simulink model "Clutchless_P2_Parallel"  (R2017b)
settings: Solver=FixedStepAuto  StartTime=0.0  StopTime=length(Speed)  FixedStep=0.01  MaxStep=0.01  RelTol=1e-3  EnableMultiTasking=on
PostLoadFcn:
  | , if any(exist('dsrtsu_mdlpostloadfcn', 'file') == [2, 3, 6]), try dsrtsu_mdlpostloadfcn('Execute', bdroot); catch fprintf('Error in PostLoadFcn (dsrtsu_mdlpostloadfcn) for model "%s":\n %s\n', bdroot, lasterr); end, end,
undefined symbols (not defined in the file): Actuators, APP1_OOR, APP2_OOR, APP_Mismatch, Brk_Flt, cal, Chassis, ClutchEngag, Clutchless_HSC, eng, Engine, EngineTorqueReal, EngOverTemp, ENGTRQ_MSMCH_Degraded_CP, ENGTRQ_MSMCH_ErrCritical_CP, ENGTRQ_MSMCH_LimpHome_CP, EngTrqMismatch, ess, ESSOverTemp, g, gb, Grade, KeyPos_Flt, lib_Actuators, lib_Chassis, lib_Clutchless_HSC, lib_EMachine_2017a, lib_Sensors_2017a, LossCAN, Machine, MCUOverTemp, mot, MotDirMismatch, motor_Trq, MotOverTemp, MotTrqMismatch, mph2ms, PRNDL_Flt, RegenFault, rho, Sensors, t_amb, time, tloop, veh, Vehicle
libraries: simulink x96, EC2_libraries x6, autolibmappedmotor x3, powerlib_meascontrol x2, CalculationGallon x1, lib_DCDC x1, lib_Differential x1, lib_HVESS x1, lib_Engine x1, lib_OBC x1, Scope_new x1, lib_Transmission x1
(part 8 of 10)

== system Clutchless_P2_Parallel/Camaro Plant Model/E-Machine/IMG Plant/Electric Machine/Torque Calculation1/max torque  ==
  cmd : Inport
  speed : Inport  Port=2
  Memory : Memory
  Peak trq max - Motoring : Lookup  InputValues=mot.plant.init.regen.trq_max.idx1_spd  Table=mot.plant.init.motor.trq_max.map  LookUpMeth=Interpolation-Use End Values  SaturateOnIntegerOverflow=on
  Peak trq max - Regen : Lookup  InputValues=mot.plant.init.regen.trq_max.idx1_spd  Table=mot.plant.init.regen.trq_max.map  LookUpMeth=Interpolation-Use End Values  SaturateOnIntegerOverflow=on
  Switch1 : Switch  SaturateOnIntegerOverflow=on
  rad/s  to RPM : Gain  Gain=30/pi
  max torque : Outport
  wires:
  Peak trq max - Regen/1 -> Switch1/3
  rad/s  to RPM/1 -> Memory/1
  Memory/1 -> Peak trq max - Regen/1, Peak trq max - Motoring/1
  Switch1/1 -> max torque/1
  cmd/1 -> Switch1/2
  speed/1 -> rad/s  to RPM/1
  Peak trq max - Motoring/1 -> Switch1/1

== system Clutchless_P2_Parallel/Camaro Plant Model/E-Machine/IMG Plant2/Thermal/Motor Thermal/Lower Limit ==
  In1 : Inport
  Constant3 : Constant  Value=Lolimit
  MinMax : MinMax  Function=max  Inputs=2
  Out1 : Outport
  wires:
  MinMax/1 -> Out1/1
  Constant3/1 -> MinMax/2
  In1/1 -> MinMax/1

== system Clutchless_P2_Parallel/Camaro Plant Model/E-Machine/IMG Plant2/Thermal1/MotInv_loop/MCUOverTemp Fault ==
  In1 : Inport
  Gain : Gain  Gain=3
  Switch : Switch  Threshold=1
  Out1 : Outport
  wires:
  Switch/1 -> Out1/1
  Gain/1 -> Switch/1
  [MCUOverTemp] -> Switch/2
  In1/1 -> Gain/1, Switch/3

== system Clutchless_P2_Parallel/Camaro Plant Model/E-Machine/IMG Plant2/Thermal1/MotInv_loop/MotorOverTempFault ==
  In1 : Inport
  Gain : Gain  Gain=2
  Switch1 : Switch  Threshold=1
  Out1 : Outport
  wires:
  Switch1/1 -> Out1/1
  Gain/1 -> Switch1/1
  [MotOverTemp] -> Switch1/2
  In1/1 -> Switch1/3, Gain/1

== system Clutchless_P2_Parallel/Camaro Plant Model/E-Machine/IMG Plant2/Thermal1/Motor Thermal/Lower Limit ==
  In1 : Inport
  Constant3 : Constant  Value=Lolimit
  MinMax : MinMax  Function=max  Inputs=2
  Out1 : Outport
  wires:
  MinMax/1 -> Out1/1
  Constant3/1 -> MinMax/2
  In1/1 -> MinMax/1

== system Clutchless_P2_Parallel/Camaro Plant Model/E-Machine/Soft MCU/Torque Calculation1/max torque /Divide by zero ==
  In1 : Inport
  Compare To Constant : simulink/Logic and Bit Operations/Compare To Constant  relop===  const=0  OutDataTypeStr=boolean
  Constant1 : Constant
  Switch2 : Switch  Criteria=u2 > Threshold
  Out1 : Outport
  wires:
  Constant1/1 -> Switch2/1
  Compare To Constant/1 -> Switch2/2
  In1/1 -> Switch2/3, Compare To Constant/1
  Switch2/1 -> Out1/1

== system Clutchless_P2_Parallel/Camaro Plant Model/E-Machine/Soft MCU/Torque Calculation1/max torque /Heat index ==
  note: Heat index calculation
  cont torque : Inport
  torque : Inport  Port=2
  Abs : Abs  SaturateOnIntegerOverflow=on
  Divide : Subsystem  mask(Divide){}
      mask Display: disp('Divide')
  Heat Energy Factor : Integrator  InitialCondition=-0.3  LimitOutput=on  UpperSaturationLimit=1  LowerSaturationLimit=-0.3
  Heating Constant : Gain  Gain=0.3/mot.plant.init.t_max_trq  SaturateOnIntegerOverflow=on  OutDataTypeStr=Inherit: Same as input  ParamDataTypeStr=Inherit: Same as input
  Saturation : Saturate  UpperLimit=1  LowerLimit=0
  Sum : Sum  Inputs=+-  SaturateOnIntegerOverflow=on  InputSameDT=on  OutDataTypeStr=Inherit: Same as first input
  motor inertia (Nms^2\rad)5 : Constant
  Heat index : Outport
  wires:
  cont torque/1 -> Divide/2(denominator)
  Abs/1 -> Sum/1
  Saturation/1 -> Heat index/1
  motor inertia (Nms^2\rad)5/1 -> Sum/2
  Divide/1(quotient) -> Abs/1
  Sum/1 -> Heating Constant/1
  Heating Constant/1 -> Heat Energy Factor/1
  Heat Energy Factor/1 -> Saturation/1
  torque/1 -> Divide/1(numerator)

== system Clutchless_P2_Parallel/Camaro Plant Model/E-Machine/Soft MCU/Torque Calculation2/max torque /Divide by zero ==
  In1 : Inport
  Compare To Constant : simulink/Logic and Bit Operations/Compare To Constant  relop===  const=0  OutDataTypeStr=boolean
  Constant1 : Constant
  Switch2 : Switch  Criteria=u2 > Threshold
  Out1 : Outport
  wires:
  Constant1/1 -> Switch2/1
  Compare To Constant/1 -> Switch2/2
  In1/1 -> Switch2/3, Compare To Constant/1
  Switch2/1 -> Out1/1

== system Clutchless_P2_Parallel/Camaro Plant Model/E-Machine/Soft MCU/Torque Calculation2/max torque /Heat index ==
  note: Heat index calculation
  cont torque : Inport
  torque : Inport  Port=2
  Abs : Abs  SaturateOnIntegerOverflow=on
  Divide : Subsystem  mask(Divide){}
      mask Display: disp('Divide')
  Heat Energy Factor : Integrator  InitialCondition=-0.3  LimitOutput=on  UpperSaturationLimit=1  LowerSaturationLimit=-0.3
  Heating Constant : Gain  Gain=0.3/mot.plant.init.t_max_trq  SaturateOnIntegerOverflow=on  OutDataTypeStr=Inherit: Same as input  ParamDataTypeStr=Inherit: Same as input
  Saturation : Saturate  UpperLimit=1  LowerLimit=0
  Sum : Sum  Inputs=+-  SaturateOnIntegerOverflow=on  InputSameDT=on  OutDataTypeStr=Inherit: Same as first input
  motor inertia (Nms^2\rad)5 : Constant
  Heat index : Outport
  wires:
  cont torque/1 -> Divide/2(denominator)
  Abs/1 -> Sum/1
  Saturation/1 -> Heat index/1
  motor inertia (Nms^2\rad)5/1 -> Sum/2
  Divide/1(quotient) -> Abs/1
  Sum/1 -> Heating Constant/1
  Heating Constant/1 -> Heat Energy Factor/1
  Heat Energy Factor/1 -> Saturation/1
  torque/1 -> Divide/1(numerator)

== system Clutchless_P2_Parallel/Camaro Plant Model/E-Machine/Soft MCU/Torque Calculation3/max torque /Divide by zero ==
  In1 : Inport
  Compare To Constant : simulink/Logic and Bit Operations/Compare To Constant  relop===  const=0  OutDataTypeStr=boolean
  Constant1 : Constant
  Switch2 : Switch  Criteria=u2 > Threshold
  Out1 : Outport
  wires:
  Constant1/1 -> Switch2/1
  Compare To Constant/1 -> Switch2/2
  In1/1 -> Switch2/3, Compare To Constant/1
  Switch2/1 -> Out1/1

== system Clutchless_P2_Parallel/Camaro Plant Model/E-Machine/Soft MCU/Torque Calculation3/max torque /Heat index ==
  note: Heat index calculation
  cont torque : Inport
  torque : Inport  Port=2
  Abs : Abs  ZeroCross=off  SaturateOnIntegerOverflow=on
  Divide : Subsystem  mask(Divide){}
      mask Display: disp('Divide')
  Heat Energy Factor : Integrator  InitialCondition=-0.3  LimitOutput=on  UpperSaturationLimit=1  LowerSaturationLimit=-0.3  ZeroCross=off
  Heating Constant : Gain  Gain=0.3/mot.plant.init.t_max_trq  SaturateOnIntegerOverflow=on  OutDataTypeStr=Inherit: Same as input  ParamDataTypeStr=Inherit: Same as input
  Saturation : Saturate  UpperLimit=1  LowerLimit=0  ZeroCross=off
  Sum : Sum  Inputs=+-  SaturateOnIntegerOverflow=on  InputSameDT=on  OutDataTypeStr=Inherit: Same as first input
  motor inertia (Nms^2\rad)5 : Constant
  Heat index : Outport
  wires:
  cont torque/1 -> Divide/2(denominator)
  Abs/1 -> Sum/1
  Saturation/1 -> Heat index/1
  motor inertia (Nms^2\rad)5/1 -> Sum/2
  Divide/1(quotient) -> Abs/1
  Sum/1 -> Heating Constant/1
  Heating Constant/1 -> Heat Energy Factor/1
  Heat Energy Factor/1 -> Saturation/1
  torque/1 -> Divide/1(numerator)

== system Clutchless_P2_Parallel/Clutchless_HSC/HSC/Camaro Fault Detection/Component Diagnostic/Engine Component Diagnostic/Override  engTrqCmd ==
  note: This subsystem is used to override the model value of a signal to a constant value
  note: Override Switch Subsystem
  In1 : Inport
  Constant : Constant  Value=50
  Multiport Switch : MultiPortSwitch  DataPortOrder=Zero-based contiguous  Inputs=2  zeroidx=on
  Signal Override Switch 0 = Use Model 1 = Use Constant : Constant
  Out1 : Outport
  wires:
  Signal Override Switch 0 = Use Model 1 = Use Constant/1 -> Multiport Switch/1
  In1/1 -> Multiport Switch/2
  Multiport Switch/1 -> Out1/1
  Constant/1 -> Multiport Switch/3

== system Clutchless_P2_Parallel/Clutchless_HSC/HSC/Camaro Fault Detection/Component Diagnostic/Engine Component Diagnostic/TorqMismatch Detection ==
  In1 : Inport
  In2 : Inport  Port=2
  In3 : Inport  Port=3
  Abs : Abs
  Add : Sum  Inputs=+-
  Bus Creator : BusCreator  Inputs=3
  Constant : Constant  Value=cal.ENGTRQ_MSMCH.ErrCritical_CP
  Constant1 : Constant  Value=50
  Constant2 : Constant  Value=cal.ENGTRQ_MSMCH.Degraded_CP
  Constant3 : Constant  Value=cal.ENGTRQ_MSMCH.LimpHome_CP
  Constant4 : Constant  Value=0
  Constant5 : Constant  Value=0
  Constant6 : Constant  Value=0
  Data Type Conversion : DataTypeConversion  OutDataTypeStr=boolean
  Data Type Conversion1 : DataTypeConversion  OutDataTypeStr=boolean
  Data Type Conversion2 : DataTypeConversion  OutDataTypeStr=boolean
  Relational Operator : RelationalOperator  OutDataTypeStr=boolean  RndMeth=Nearest
  Relational Operator1 : RelationalOperator  Operator=>  OutDataTypeStr=boolean  RndMeth=Nearest
  Relational Operator2 : RelationalOperator  Operator=>  OutDataTypeStr=boolean  RndMeth=Nearest
  Switch : Switch  Threshold=1
  Terminator{,1..3} (4 alike) : Terminator
  Unit Delay : UnitDelay  Commented=through  SampleTime=-1
  Unit Delay1 : UnitDelay  Commented=through  SampleTime=-1
  "Zero " : Constant  Value=0
  Eng_Torque_Mismch : Outport
  wires:
  Constant1/1 -> Terminator3/1
  In1/1 -> Unit Delay/1
  In2/1 -> Unit Delay1/1
  "Zero "/1 -> Switch/3
  In3/1 -> Switch/2
  Unit Delay/1 -> Add/1
  Constant/1 -> Relational Operator/2
  Add/1 -> Abs/1
  Relational Operator/1 -> Switch/1
  Switch/1 -> Relational Operator2/1, Relational Operator1/1, Terminator/1  "Eng_Torque_Mismch_Critical"
  Constant2/1 -> Relational Operator1/2
  Constant3/1 -> Relational Operator2/2
  Relational Operator1/1 -> Terminator1/1  "Eng_Torque_Mismch_Degrad"
  Relational Operator2/1 -> Terminator2/1  "Eng_Torque_Mismch_Limp"
  Bus Creator/1 -> Eng_Torque_Mismch/1
  Unit Delay1/1 -> Add/2
  Abs/1 -> Relational Operator/1
  Constant4/1 -> Data Type Conversion/1  "Eng_Torque_Mismch_Critical"
  Constant6/1 -> Data Type Conversion2/1  "Eng_Torque_Mismch_Limp"
  Constant5/1 -> Data Type Conversion1/1  "Eng_Torque_Mismch_Degrad"
  Data Type Conversion/1 -> Bus Creator/1  "Eng_Torque_Mismch_Critical"
  Data Type Conversion1/1 -> Bus Creator/2  "Eng_Torque_Mismch_Degrad"
  Data Type Conversion2/1 -> Bus Creator/3  "Eng_Torque_Mismch_Limp"

== system Clutchless_P2_Parallel/Clutchless_HSC/HSC/Camaro Fault Detection/Input Conversions/BMS_Conversions/Override  BMS_gdf 0_1 ==
  note: Override Switch Subsystem
  note: This subsystem is used to override the model value of a signal to a constant value
  In1 : Inport
  Multiport Switch : MultiPortSwitch  DataPortOrder=Zero-based contiguous  Inputs=2  zeroidx=on
  Override Value : Constant  Value=0  OutDataTypeStr=double
  Signal Override Switch 0 = Use Model 1 = Use Constant : Constant
  Out1 : Outport
  wires:
  Override Value/1 -> Multiport Switch/3
  Multiport Switch/1 -> Out1/1
  In1/1 -> Multiport Switch/2
  Signal Override Switch 0 = Use Model 1 = Use Constant/1 -> Multiport Switch/1

== system Clutchless_P2_Parallel/Clutchless_HSC/HSC/Camaro Fault Detection/Input Conversions/BMS_Conversions/Override  closeContactorsCmd ==
  note: This subsystem is used to override the model value of a signal to a constant value
  note: Override Switch Subsystem
  In1 : Inport
  Multiport Switch : MultiPortSwitch  DataPortOrder=Zero-based contiguous  Inputs=2  zeroidx=on
  Override Value : Constant  Value=0  OutDataTypeStr=double
  Signal Override Switch 0 = Use Model 1 = Use Constant : Constant  Value=0
  Out1 : Outport
  wires:
  Signal Override Switch 0 = Use Model 1 = Use Constant/1 -> Multiport Switch/1
  In1/1 -> Multiport Switch/2
  Multiport Switch/1 -> Out1/1
  Override Value/1 -> Multiport Switch/3

== system Clutchless_P2_Parallel/Clutchless_HSC/HSC/Camaro Fault Detection/Input Conversions/BMS_Conversions/Override  contactorsClsd ==
  note: This subsystem is used to override the model value of a signal to a constant value
  note: Override Switch Subsystem
  In1 : Inport
  Multiport Switch : MultiPortSwitch  DataPortOrder=Zero-based contiguous  Inputs=2  zeroidx=on
  Override Value : Constant  Value=0  OutDataTypeStr=double
  Signal Override Switch 0 = Use Model 1 = Use Constant : Constant  Value=0
  Out1 : Outport
  wires:
  Signal Override Switch 0 = Use Model 1 = Use Constant/1 -> Multiport Switch/1
  In1/1 -> Multiport Switch/2
  Multiport Switch/1 -> Out1/1
  Override Value/1 -> Multiport Switch/3

== system Clutchless_P2_Parallel/Clutchless_HSC/HSC/Camaro Fault Detection/Input Conversions/BMS_Conversions/Override  essCur_A ==
  note: Override Switch Subsystem
  note: This subsystem is used to override the model value of a signal to a constant value
  In1 : Inport
  Multiport Switch : MultiPortSwitch  DataPortOrder=Zero-based contiguous  Inputs=2  zeroidx=on
  Override Value : Constant  Value=0  OutDataTypeStr=double
  Signal Override Switch 0 = Use Model 1 = Use Constant : Constant  Value=0
  Out1 : Outport
  wires:
  Override Value/1 -> Multiport Switch/3
  Multiport Switch/1 -> Out1/1
  In1/1 -> Multiport Switch/2
  Signal Override Switch 0 = Use Model 1 = Use Constant/1 -> Multiport Switch/1

== system Clutchless_P2_Parallel/Clutchless_HSC/HSC/Camaro Fault Detection/Input Conversions/BMS_Conversions/Override  essSOC_0_1 ==
  note: This subsystem is used to override the model value of a signal to a constant value
  note: Override Switch Subsystem
  In1 : Inport
  Multiport Switch : MultiPortSwitch  DataPortOrder=Zero-based contiguous  Inputs=2  zeroidx=on
  Override Value : Constant  Value=0  OutDataTypeStr=double
  Signal Override Switch 0 = Use Model 1 = Use Constant : Constant  Value=0
  Out1 : Outport
  wires:
  Signal Override Switch 0 = Use Model 1 = Use Constant/1 -> Multiport Switch/1
  In1/1 -> Multiport Switch/2
  Multiport Switch/1 -> Out1/1
  Override Value/1 -> Multiport Switch/3

== system Clutchless_P2_Parallel/Clutchless_HSC/HSC/Camaro Fault Detection/Input Conversions/BMS_Conversions/Override  essTemp_C ==
  note: This subsystem is used to override the model value of a signal to a constant value
  note: Override Switch Subsystem
  In1 : Inport
  Multiport Switch : MultiPortSwitch  DataPortOrder=Zero-based contiguous  Inputs=2  zeroidx=on
  Override Value : Constant  Value=0  OutDataTypeStr=double
  Signal Override Switch 0 = Use Model 1 = Use Constant : Constant
  Out1 : Outport
  wires:
  Signal Override Switch 0 = Use Model 1 = Use Constant/1 -> Multiport Switch/1
  In1/1 -> Multiport Switch/2
  Multiport Switch/1 -> Out1/1
  Override Value/1 -> Multiport Switch/3

== system Clutchless_P2_Parallel/Clutchless_HSC/HSC/Camaro Fault Detection/Input Conversions/BMS_Conversions/Override  hvBattVolt_V ==
  note: This subsystem is used to override the model value of a signal to a constant value
  note: Override Switch Subsystem
  In1 : Inport
  Multiport Switch : MultiPortSwitch  DataPortOrder=Zero-based contiguous  Inputs=2  zeroidx=on
  Override Value : Constant  Value=0  OutDataTypeStr=double
  Signal Override Switch 0 = Use Model 1 = Use Constant : Constant  Value=0
  Out1 : Outport
  wires:
  Signal Override Switch 0 = Use Model 1 = Use Constant/1 -> Multiport Switch/1
  In1/1 -> Multiport Switch/2
  Multiport Switch/1 -> Out1/1
  Override Value/1 -> Multiport Switch/3

== system Clutchless_P2_Parallel/Clutchless_HSC/HSC/Camaro Fault Detection/Input Conversions/BMS_Conversions/Override  hvBusVolt_V ==
  note: Override Switch Subsystem
  note: This subsystem is used to override the model value of a signal to a constant value
  In1 : Inport
  Multiport Switch : MultiPortSwitch  DataPortOrder=Zero-based contiguous  Inputs=2  zeroidx=on
  Override Value : Constant  Value=0  OutDataTypeStr=double
  Signal Override Switch 0 = Use Model 1 = Use Constant : Constant  Value=0
  Out1 : Outport
  wires:
  Override Value/1 -> Multiport Switch/3
  Multiport Switch/1 -> Out1/1
  In1/1 -> Multiport Switch/2
  Signal Override Switch 0 = Use Model 1 = Use Constant/1 -> Multiport Switch/1

== system Clutchless_P2_Parallel/Clutchless_HSC/HSC/Camaro Fault Detection/Input Conversions/BMS_Conversions/Override  rollingAliveCnt [1_3] ==
  note: Override Switch Subsystem
  note: This subsystem is used to override the model value of a signal to a constant value
  In1 : Inport
  Multiport Switch : MultiPortSwitch  DataPortOrder=Zero-based contiguous  Inputs=2  zeroidx=on
  Override Value : Constant  Value=0  OutDataTypeStr=double
  Signal Override Switch 0 = Use Model 1 = Use Constant : Constant  Value=0
  Out1 : Outport
  wires:
  Override Value/1 -> Multiport Switch/3
  Multiport Switch/1 -> Out1/1
  In1/1 -> Multiport Switch/2
  Signal Override Switch 0 = Use Model 1 = Use Constant/1 -> Multiport Switch/1

== system Clutchless_P2_Parallel/Clutchless_HSC/HSC/Camaro Fault Detection/Input Conversions/BMS_Conversions/Override Fehler_HS_offen ==
  note: This subsystem is used to override the model value of a signal to a constant value
  note: Override Switch Subsystem
  In1 : Inport
  Multiport Switch : MultiPortSwitch  DataPortOrder=Zero-based contiguous  Inputs=2  zeroidx=on
  Override Value : Constant  Value=0  OutDataTypeStr=double
  Signal Override Switch 0 = Use Model 1 = Use Constant : Constant
  Out1 : Outport
  wires:
  Signal Override Switch 0 = Use Model 1 = Use Constant/1 -> Multiport Switch/1
  In1/1 -> Multiport Switch/2
  Multiport Switch/1 -> Out1/1
  Override Value/1 -> Multiport Switch/3

== system Clutchless_P2_Parallel/Clutchless_HSC/HSC/Camaro Fault Detection/Input Conversions/BMS_Conversions/Override Fehler_HS_verschweisst ==
  note: Override Switch Subsystem
  note: This subsystem is used to override the model value of a signal to a constant value
  In1 : Inport
  Multiport Switch : MultiPortSwitch  DataPortOrder=Zero-based contiguous  Inputs=2  zeroidx=on
  Override Value : Constant  Value=0  OutDataTypeStr=double
  Signal Override Switch 0 = Use Model 1 = Use Constant : Constant
  Out1 : Outport
  wires:
  Override Value/1 -> Multiport Switch/3
  Multiport Switch/1 -> Out1/1
  In1/1 -> Multiport Switch/2
  Signal Override Switch 0 = Use Model 1 = Use Constant/1 -> Multiport Switch/1

== system Clutchless_P2_Parallel/Clutchless_HSC/HSC/Camaro Fault Detection/Input Conversions/DriverInput_Conversions/Override  KeyPos [0_3] ==
  note: Override Switch Subsystem
  note: This subsystem is used to override the model value of a signal to a constant value
  In1 : Inport
  Multiport Switch : MultiPortSwitch  DataPortOrder=Zero-based contiguous  Inputs=2  zeroidx=on
  Override Value : Constant  Value=0  OutDataTypeStr=double
  Signal Override Switch 0 = Use Model 1 = Use Constant : Constant  Value=0
  Out1 : Outport
  wires:
  Override Value/1 -> Multiport Switch/3
  Multiport Switch/1 -> Out1/1
  In1/1 -> Multiport Switch/2
  Signal Override Switch 0 = Use Model 1 = Use Constant/1 -> Multiport Switch/1

== system Clutchless_P2_Parallel/Clutchless_HSC/HSC/Camaro Fault Detection/Input Conversions/DriverInput_Conversions/Override APP (%) ==
  note: Override Switch Subsystem
  note: This subsystem is used to override the model value of a signal to a constant value
  In1 : Inport
  Multiport Switch : MultiPortSwitch  DataPortOrder=Zero-based contiguous  Inputs=2  zeroidx=on
  Override Value : Constant  Value=0  OutDataTypeStr=double
  Signal Override Switch 0 = Use Model 1 = Use Constant : Constant  Value=0
  Out1 : Outport
  wires:
  Override Value/1 -> Multiport Switch/3
  Multiport Switch/1 -> Out1/1
  In1/1 -> Multiport Switch/2
  Signal Override Switch 0 = Use Model 1 = Use Constant/1 -> Multiport Switch/1

== system Clutchless_P2_Parallel/Clutchless_HSC/HSC/Camaro Fault Detection/Input Conversions/DriverInput_Conversions/Override APP (%)1 ==
  note: This subsystem is used to override the model value of a signal to a constant value
  note: Override Switch Subsystem
  In1 : Inport
  Multiport Switch : MultiPortSwitch  DataPortOrder=Zero-based contiguous  Inputs=2  zeroidx=on
  Override Value : Constant  Value=0  OutDataTypeStr=double
  Signal Override Switch 0 = Use Model 1 = Use Constant : Constant  Value=0
  Out1 : Outport
  wires:
  Signal Override Switch 0 = Use Model 1 = Use Constant/1 -> Multiport Switch/1
  In1/1 -> Multiport Switch/2
  Multiport Switch/1 -> Out1/1
  Override Value/1 -> Multiport Switch/3

== system Clutchless_P2_Parallel/Clutchless_HSC/HSC/Camaro Fault Detection/Input Conversions/DriverInput_Conversions/Override BPP (%) ==
  note: This subsystem is used to override the model value of a signal to a constant value
  note: Override Switch Subsystem
  In1 : Inport
  Multiport Switch : MultiPortSwitch  DataPortOrder=Zero-based contiguous  Inputs=2  zeroidx=on
  Override Value : Constant  Value=0  OutDataTypeStr=double
  Signal Override Switch 0 = Use Model 1 = Use Constant : Constant  Value=0
  Out1 : Outport
  wires:
  Signal Override Switch 0 = Use Model 1 = Use Constant/1 -> Multiport Switch/1
  In1/1 -> Multiport Switch/2
  Multiport Switch/1 -> Out1/1
  Override Value/1 -> Multiport Switch/3

== system Clutchless_P2_Parallel/Clutchless_HSC/HSC/Camaro Fault Detection/Input Conversions/DriverInput_Conversions/Override PRNDL ==
  note: Override Switch Subsystem
  note: This subsystem is used to override the model value of a signal to a constant value
  In1 : Inport
  Multiport Switch : MultiPortSwitch  DataPortOrder=Zero-based contiguous  Inputs=2  zeroidx=on
  Override Value : Constant  Value=0  OutDataTypeStr=double
  Signal Override Switch 0 = Use Model 1 = Use Constant : Constant  Value=0
  Out1 : Outport
  wires:
  Override Value/1 -> Multiport Switch/3
  Multiport Switch/1 -> Out1/1
  In1/1 -> Multiport Switch/2
  Signal Override Switch 0 = Use Model 1 = Use Constant/1 -> Multiport Switch/1

== system Clutchless_P2_Parallel/Clutchless_HSC/HSC/Camaro Fault Detection/Input Conversions/DriverInput_Conversions/Override Regen ==
  note: Override Switch Subsystem
  note: This subsystem is used to override the model value of a signal to a constant value
  In1 : Inport
  Multiport Switch : MultiPortSwitch  DataPortOrder=Zero-based contiguous  Inputs=2  zeroidx=on
  Override Value : Constant  Value=0  OutDataTypeStr=double
  Signal Override Switch 0 = Use Model 1 = Use Constant : Constant  Value=0
  Out1 : Outport
  wires:
  Override Value/1 -> Multiport Switch/3
  Multiport Switch/1 -> Out1/1
  In1/1 -> Multiport Switch/2
  Signal Override Switch 0 = Use Model 1 = Use Constant/1 -> Multiport Switch/1

== system Clutchless_P2_Parallel/Clutchless_HSC/HSC/Camaro Fault Detection/Input Conversions/DriverInput_Conversions/Override V [mph] ==
  note: This subsystem is used to override the model value of a signal to a constant value
  note: Override Switch Subsystem
  In1 : Inport
  Multiport Switch : MultiPortSwitch  DataPortOrder=Zero-based contiguous  Inputs=2  zeroidx=on
  Override Value : Constant  Value=0  OutDataTypeStr=double
  Signal Override Switch 0 = Use Model 1 = Use Constant : Constant  Value=0
  Out1 : Outport
  wires:
  Signal Override Switch 0 = Use Model 1 = Use Constant/1 -> Multiport Switch/1
  In1/1 -> Multiport Switch/2
  Multiport Switch/1 -> Out1/1
  Override Value/1 -> Multiport Switch/3

== system Clutchless_P2_Parallel/Clutchless_HSC/HSC/Camaro Fault Detection/Input Conversions/ECM_Conversions/Override  ECMTrqCmd_Nm ==
  note: This subsystem is used to override the model value of a signal to a constant value
  note: Override Switch Subsystem
  In1 : Inport
  Multiport Switch : MultiPortSwitch  DataPortOrder=Zero-based contiguous  Inputs=2  zeroidx=on
  Override Value : Constant  Value=0  OutDataTypeStr=double
  Signal Override Switch 0 = Use Model 1 = Use Constant : Constant  Value=0
  Out1 : Outport
  wires:
  Signal Override Switch 0 = Use Model 1 = Use Constant/1 -> Multiport Switch/1
  In1/1 -> Multiport Switch/2
  Multiport Switch/1 -> Out1/1
  Override Value/1 -> Multiport Switch/3

== system Clutchless_P2_Parallel/Clutchless_HSC/HSC/Camaro Fault Detection/Input Conversions/ECM_Conversions/Override  ECMrollingAliveCnt ==
  note: Override Switch Subsystem
  note: This subsystem is used to override the model value of a signal to a constant value
  In1 : Inport
  Multiport Switch : MultiPortSwitch  DataPortOrder=Zero-based contiguous  Inputs=2  zeroidx=on
  Override Value : Constant  Value=0  OutDataTypeStr=double
  Signal Override Switch 0 = Use Model 1 = Use Constant : Constant  Value=0
  Out1 : Outport
  wires:
  Override Value/1 -> Multiport Switch/3
  Multiport Switch/1 -> Out1/1
  In1/1 -> Multiport Switch/2
  Signal Override Switch 0 = Use Model 1 = Use Constant/1 -> Multiport Switch/1

== system Clutchless_P2_Parallel/Clutchless_HSC/HSC/Camaro Fault Detection/Input Conversions/ECM_Conversions/Override  EngActStdyStTorq_Nm ==
  note: Override Switch Subsystem
  note: This subsystem is used to override the model value of a signal to a constant value
  In1 : Inport
  Multiport Switch : MultiPortSwitch  DataPortOrder=Zero-based contiguous  Inputs=2  zeroidx=on
  Override Value : Constant  Value=0  OutDataTypeStr=double
  Signal Override Switch 0 = Use Model 1 = Use Constant : Constant  Value=0
  Out1 : Outport
  wires:
  Override Value/1 -> Multiport Switch/3
  Multiport Switch/1 -> Out1/1
  In1/1 -> Multiport Switch/2
  Signal Override Switch 0 = Use Model 1 = Use Constant/1 -> Multiport Switch/1

== system Clutchless_P2_Parallel/Clutchless_HSC/HSC/Camaro Fault Detection/Input Conversions/ECM_Conversions/Override  EngRunAtv ==
  note: This subsystem is used to override the model value of a signal to a constant value
  note: Override Switch Subsystem
  In1 : Inport
  Multiport Switch : MultiPortSwitch  DataPortOrder=Zero-based contiguous  Inputs=2  zeroidx=on
  Override Value : Constant  Value=0  OutDataTypeStr=double
  Signal Override Switch 0 = Use Model 1 = Use Constant : Constant  Value=0
  Out1 : Outport
  wires:
  Signal Override Switch 0 = Use Model 1 = Use Constant/1 -> Multiport Switch/1
  In1/1 -> Multiport Switch/2
  Multiport Switch/1 -> Out1/1
  Override Value/1 -> Multiport Switch/3

== system Clutchless_P2_Parallel/Clutchless_HSC/HSC/Camaro Fault Detection/Input Conversions/ECM_Conversions/Override  EngineSpeed_rpm ==
  note: This subsystem is used to override the model value of a signal to a constant value
  note: Override Switch Subsystem
  In1 : Inport
  Multiport Switch : MultiPortSwitch  DataPortOrder=Zero-based contiguous  Inputs=2  zeroidx=on
  Override Value : Constant  Value=0  OutDataTypeStr=double
  Signal Override Switch 0 = Use Model 1 = Use Constant : Constant  Value=0
  Out1 : Outport
  wires:
  Signal Override Switch 0 = Use Model 1 = Use Constant/1 -> Multiport Switch/1
  In1/1 -> Multiport Switch/2
  Multiport Switch/1 -> Out1/1
  Override Value/1 -> Multiport Switch/3

== system Clutchless_P2_Parallel/Clutchless_HSC/HSC/Camaro Fault Detection/Input Conversions/ECM_Conversions/Override  Engine_Temp[DegC] ==
  note: Override Switch Subsystem
  note: This subsystem is used to override the model value of a signal to a constant value
  In1 : Inport
  Multiport Switch : MultiPortSwitch  DataPortOrder=Zero-based contiguous  Inputs=2  zeroidx=on
  Override Value : Constant  Value=0  OutDataTypeStr=double
  Signal Override Switch 0 = Use Model 1 = Use Constant : Constant  Value=0
  Out1 : Outport
  wires:
  Override Value/1 -> Multiport Switch/3
  Multiport Switch/1 -> Out1/1
  In1/1 -> Multiport Switch/2
  Signal Override Switch 0 = Use Model 1 = Use Constant/1 -> Multiport Switch/1

== system Clutchless_P2_Parallel/Clutchless_HSC/HSC/Camaro Fault Detection/Input Conversions/TCM_Conversions/Override  LockupCmd ==
  note: This subsystem is used to override the model value of a signal to a constant value
  note: Override Switch Subsystem
  In1 : Inport
  Multiport Switch : MultiPortSwitch  DataPortOrder=Zero-based contiguous  Inputs=2  zeroidx=on
  Override Value : Constant  Value=0  OutDataTypeStr=double
  Signal Override Switch 0 = Use Model 1 = Use Constant : Constant  Value=0
  Out1 : Outport
  wires:
  Signal Override Switch 0 = Use Model 1 = Use Constant/1 -> Multiport Switch/1
  In1/1 -> Multiport Switch/2
  Multiport Switch/1 -> Out1/1
  Override Value/1 -> Multiport Switch/3

== system Clutchless_P2_Parallel/Clutchless_HSC/HSC/Camaro Fault Detection/Input Conversions/TCM_Conversions/Override  LvrPosTrnsShft  ==
  note: This subsystem is used to override the model value of a signal to a constant value
  note: Override Switch Subsystem
  In1 : Inport
  Multiport Switch : MultiPortSwitch  DataPortOrder=Zero-based contiguous  Inputs=2  zeroidx=on
  Override Value : Constant  Value=0  OutDataTypeStr=double
  Signal Override Switch 0 = Use Model 1 = Use Constant : Constant  Value=0
  Out1 : Outport
  wires:
  Signal Override Switch 0 = Use Model 1 = Use Constant/1 -> Multiport Switch/1
  In1/1 -> Multiport Switch/2
  Multiport Switch/1 -> Out1/1
  Override Value/1 -> Multiport Switch/3

== system Clutchless_P2_Parallel/Clutchless_HSC/HSC/Camaro Fault Detection/Input Conversions/TCM_Conversions/Override  TransEstGear ==
  note: This subsystem is used to override the model value of a signal to a constant value
  note: Override Switch Subsystem
  In1 : Inport
  Multiport Switch : MultiPortSwitch  DataPortOrder=Zero-based contiguous  Inputs=2  zeroidx=on
  Override Value : Constant  Value=0  OutDataTypeStr=double
  Signal Override Switch 0 = Use Model 1 = Use Constant : Constant  Value=0
  Out1 : Outport
  wires:
  Signal Override Switch 0 = Use Model 1 = Use Constant/1 -> Multiport Switch/1
  In1/1 -> Multiport Switch/2
  Multiport Switch/1 -> Out1/1
  Override Value/1 -> Multiport Switch/3

== system Clutchless_P2_Parallel/Clutchless_HSC/HSC/Camaro Fault Detection/Input Conversions/TCM_Conversions/Override  rollingAliveCnt [123] ==
  note: This subsystem is used to override the model value of a signal to a constant value
  note: Override Switch Subsystem
  In1 : Inport
  Multiport Switch : MultiPortSwitch  DataPortOrder=Zero-based contiguous  Inputs=2  zeroidx=on
  Override Value : Constant  Value=0  OutDataTypeStr=double
  Signal Override Switch 0 = Use Model 1 = Use Constant : Constant  Value=0
  Out1 : Outport
  wires:
  Signal Override Switch 0 = Use Model 1 = Use Constant/1 -> Multiport Switch/1
  In1/1 -> Multiport Switch/2
  Multiport Switch/1 -> Out1/1
  Override Value/1 -> Multiport Switch/3

== system Clutchless_P2_Parallel/Clutchless_HSC/HSC/Camaro Fault Detection/Input Conversions/TCM_Conversions/TCM_RollinAliveCounter ==
  Constant : Constant  Value=0
  Constant8 : Constant
  Rolling Alive Counter1 : Stateflow chart  TreatAsAtomicUnit=on
  Switch1 : Switch  Criteria=u2 > Threshold
  Out1 : Outport
  wires:
  Constant/1 -> [TCM_CAN_fault]
  Switch1/1 -> Out1/1  "TCMRollingAliveCnt [0 1 2 3]"
  [TCM_CAN_fault] -> Switch1/2
  Rolling Alive Counter1/1(RollingAliveCnt) -> Switch1/3
  Constant8/1 -> Switch1/1

== system Clutchless_P2_Parallel/Clutchless_HSC/HSC/Camaro Fault Detection/Signal Diagnostic/Driver Signal Diagnostic/APP_Crosscheck ==
  In1 : Inport
  In2 : Inport  Port=2
  Abs : Abs
  Compare To Constant : simulink/Logic and Bit Operations/Compare To Constant  relop=<=  const=0.5  OutDataTypeStr=boolean
  Sum : Sum  Inputs=+-
  Out1 : Outport
  wires:
  Sum/1 -> Abs/1
  Abs/1 -> Compare To Constant/1
  In1/1 -> Sum/1
  In2/1 -> Sum/2
  Compare To Constant/1 -> Out1/1  "Drv_APP_Agree"

== system Clutchless_P2_Parallel/Clutchless_HSC/HSC/Camaro Fault Detection/Signal Diagnostic/Driver Signal Diagnostic/BrakeFailureDetection ==
  BPP : Inport
  VehSpeed : Inport  Port=2
  Trigger : TriggerPort  VariantControl=Variant  PortDimensions=1
  Chart : Stateflow chart  Commented=on  TreatAsAtomicUnit=on
  Compare To Constant : simulink/Logic and Bit Operations/Compare To Constant  relop=>  const=0  OutDataTypeStr=boolean
  Compare To Constant1 : simulink/Logic and Bit Operations/Compare To Constant  relop=>  const=0.5  OutDataTypeStr=boolean
  Detect Change : simulink/Logic and Bit Operations/Detect Change  vinit=0  InputProcessing=Inherited  OutDataTypeStr=boolean
  Detect Increase : simulink/Logic and Bit Operations/Detect Increase  vinit=0.0  InputProcessing=Inherited  OutDataTypeStr=boolean
  Logical Operator : Logic  Operator=NOT  AllPortsSameDT=off  OutDataTypeStr=boolean
  Logical Operator1 : Logic  AllPortsSameDT=off  OutDataTypeStr=boolean
  Logical Operator2 : Logic  Operator=OR  AllPortsSameDT=off  OutDataTypeStr=boolean
  Logical Operator3 : Logic  AllPortsSameDT=off  OutDataTypeStr=boolean
  Unit Delay : UnitDelay  SampleTime=-1
  Unit Delay1 : UnitDelay  SampleTime=-1
  DecelFail : Outport
  wires:
  VehSpeed/1 -> Unit Delay1/1, Detect Change/1, Detect Increase/1
  Detect Change/1 -> Logical Operator/1
  Compare To Constant/1 -> Logical Operator1/1
  Compare To Constant1/1 -> Logical Operator1/2
  BPP/1 -> Unit Delay/1
  Logical Operator1/1 -> Logical Operator3/1
  Detect Increase/1 -> Logical Operator2/1  "Increase"
  Logical Operator/1 -> Logical Operator2/2  "Unchange"
  Unit Delay/1 -> Compare To Constant/1
  Unit Delay1/1 -> Compare To Constant1/1
  Logical Operator2/1 -> Logical Operator3/2
  Logical Operator3/1 -> DecelFail/1

== system Clutchless_P2_Parallel/Clutchless_HSC/HSC/Camaro Fault Detection/Signal Diagnostic/Driver Signal Diagnostic/Latch ==
  In1 : Inport
  In2 : Inport  Port=2
  Memory : Memory
  NOT : Logic  Operator=NOT  OutDataTypeStr=boolean
  OR : Logic  OutDataTypeStr=boolean
  OR1 : Logic  Operator=OR  OutDataTypeStr=boolean
  Drv_APP_Agree : Outport
  wires:
  In1/1 -> OR1/1
  OR/1 -> OR1/2
  OR1/1 -> Drv_APP_Agree/1, Memory/1
  NOT/1 -> OR/1
  Memory/1 -> OR/2
  In2/1 -> NOT/1

== system Clutchless_P2_Parallel/Clutchless_HSC/HSC/Camaro Fault Detection/Signal Diagnostic/Driver Signal Diagnostic/Latch1 ==
  In1 : Inport
  In2 : Inport  Port=2
  Memory : Memory
  NOT : Logic  Operator=NOT  OutDataTypeStr=boolean
  OR : Logic  OutDataTypeStr=boolean
  OR1 : Logic  Operator=OR  OutDataTypeStr=boolean
  Out1 : Outport
  wires:
  In2/1 -> NOT/1
  Memory/1 -> OR/2
  NOT/1 -> OR/1
  OR1/1 -> Memory/1, Out1/1
  OR/1 -> OR1/2
  In1/1 -> OR1/1

== system Clutchless_P2_Parallel/Clutchless_HSC/HSC/Camaro Fault Detection/Signal Diagnostic/ESS Signal Diagnostic/Contactors status check ==
  note: Note: Contactors don't close when commanded
  In1 : Inport
  In2 : Inport  Port=2
  In3 : Inport  Port=3
  " " : simulink/Logic and Bit Operations/Compare To Constant  relop=>  const=0.5  OutDataTypeStr=boolean
  Abs : Abs
  Logical Operator : Logic  Operator=OR  AllPortsSameDT=off  OutDataTypeStr=boolean
  Sum : Sum  Inputs=+-
  Out1 : Outport
  wires:
  " "/1 -> Logical Operator/1  "BMS_contactorsFailed_SigValid"
  In3/1 -> Logical Operator/2
  In2/1 -> Sum/2
  Abs/1 -> " "/1
  Sum/1 -> Abs/1
  Logical Operator/1 -> Out1/1  "BMS_contactorsFailed_Detected"
  In1/1 -> Sum/1

== system Clutchless_P2_Parallel/Clutchless_HSC/HSC/Camaro Fault Detection/Signal Diagnostic/ESS Signal Diagnostic/ESS SOC Validity Check ==
  In1 : Inport
  Constant1 : Constant
  essSOCValidity_Check : Subsystem
  essSOC_0_1Range : Stateflow chart  TreatAsAtomicUnit=on
  Out1 : Outport
  Out2 : Outport  Port=2
  wires:
  essSOCValidity_Check/1(Out1) -> Out1/1  "BMS_essSOC_0_1_SigValid"
  In1/1 -> essSOC_0_1Range/2(signalValue)
  Constant1/1 -> essSOC_0_1Range/1(clearFaults)
  essSOC_0_1Range/1(essSOCRange) -> Out2/1, essSOCValidity_Check/1(In1)

== system Clutchless_P2_Parallel/Clutchless_HSC/HSC/Camaro Fault Detection/Signal Diagnostic/ESS Signal Diagnostic/ESS Temp Validity Check ==
  In1 : Inport
  Constant : Constant
  essTsignalRange : Stateflow chart  TreatAsAtomicUnit=on
  essTsignalValidity_Check : Subsystem
  Out1 : Outport
  Out2 : Outport  Port=2
  wires:
  Constant/1 -> essTsignalRange/1(clearFaults)
  essTsignalValidity_Check/1(Out1) -> Out1/1  "BMS_essTemp_[degC]_SigValid"
  essTsignalRange/1(essTempRange) -> Out2/1, essTsignalValidity_Check/1(In1)  "essTempRange[0_4]"
  In1/1 -> essTsignalRange/2(signalValue)

== system Clutchless_P2_Parallel/Clutchless_HSC/HSC/Camaro Fault Detection/Signal Diagnostic/ESS Signal Diagnostic/Max charging voltage fault detect ==
  note: Note: When the ESS receives the energy from grid or regenerative braking,
      | the charging voltage to the inverter can not be bigger than 419V, otherwise the MCU will set to fault
  In1 : Inport
  " " : simulink/Logic and Bit Operations/Compare To Constant  relop=>  const=419  OutDataTypeStr=boolean
  Abs : Abs
  Compare To Zero : simulink/Logic and Bit Operations/Compare To Zero  relop=<  OutDataTypeStr=boolean
  Logical Operator : Logic  AllPortsSameDT=off  OutDataTypeStr=boolean
  Out1 : Outport
  wires:
  Compare To Zero/1 -> Logical Operator/2
  In1/1 -> Abs/1, Compare To Zero/1
  " "/1 -> Logical Operator/1
  Logical Operator/1 -> Out1/1
  Abs/1 -> " "/1

== system Clutchless_P2_Parallel/Clutchless_HSC/HSC/Camaro Fault Detection/Signal Diagnostic/ESS Signal Diagnostic/Rolling Alive Counter Detection ==
  In1 : Inport
  Chart : Stateflow chart  TreatAsAtomicUnit=on
  Constant : Constant  Value=0.01
  Constant1 : Constant  Value=0.01
  Detect Change : simulink/Logic and Bit Operations/Detect Change  vinit=1  InputProcessing=Inherited  OutDataTypeStr=boolean
  Out1 : Outport
  wires:
  Constant/1 -> Chart/2(CycleTime)
  Chart/1(flag) -> Out1/1
  Detect Change/1 -> Chart/1(PulseDetect)
  In1/1 -> Detect Change/1
  Constant1/1 -> Chart/3(tloop)

== system Clutchless_P2_Parallel/Clutchless_HSC/HSC/Camaro Fault Detection/Signal Diagnostic/ESS Signal Diagnostic/Validity Check ==
  In1 : Inport
  " Normal Operation" : simulink/Logic and Bit Operations/Compare To Constant  relop===  const=1  OutDataTypeStr=boolean
  Below Normal Operation : simulink/Logic and Bit Operations/Compare To Constant  relop===  const=0  OutDataTypeStr=boolean
  Logical Operator : Logic  Operator=OR  AllPortsSameDT=off  OutDataTypeStr=boolean
  Out1 : Outport
  wires:
  Logical Operator/1 -> Out1/1  "BMSgdf_SigValid"
  " Normal Operation"/1 -> Logical Operator/2
  Below Normal Operation/1 -> Logical Operator/1
  In1/1 -> " Normal Operation"/1, Below Normal Operation/1

== system Clutchless_P2_Parallel/Clutchless_HSC/HSC/Camaro Fault Detection/Signal Diagnostic/Engine Signal Diagnostic/EngTempValidity_Check ==
  In1 : Inport
  Above Normal Operation : simulink/Logic and Bit Operations/Compare To Constant  relop===  const=3  OutDataTypeStr=boolean
  Logical Operator1 : Logic  Operator=NOT  AllPortsSameDT=off  OutDataTypeStr=boolean
  Out1 : Outport
  wires:
  In1/1 -> Above Normal Operation/1
  Above Normal Operation/1 -> Logical Operator1/1
  Logical Operator1/1 -> Out1/1

== system Clutchless_P2_Parallel/Clutchless_HSC/HSC/Camaro Fault Detection/Signal Diagnostic/Engine Signal Diagnostic/Rolling Alive Counter Detection1 ==
  In1 : Inport
  Chart : Stateflow chart  TreatAsAtomicUnit=on
  Constant : Constant  Value=0.01
  Detect Change : simulink/Logic and Bit Operations/Detect Change  vinit=1  InputProcessing=Inherited  OutDataTypeStr=boolean
  Out1 : Outport
  wires:
  In1/1 -> Detect Change/1
  Detect Change/1 -> Chart/1(PulseDetect)
  Chart/1(flag) -> Out1/1
  Constant/1 -> Chart/2(CycleTime)

== system Clutchless_P2_Parallel/Clutchless_HSC/HSC/Camaro Fault Detection/Signal Diagnostic/Transmission Signal Diagnostic/Rolling Alive Counter Detection ==
  In1 : Inport
  Chart : Stateflow chart  TreatAsAtomicUnit=on
  Constant : Constant  Value=0.01
  Detect Change : simulink/Logic and Bit Operations/Detect Change  vinit=1  InputProcessing=Inherited  OutDataTypeStr=boolean
  Out1 : Outport
  wires:
  In1/1 -> Detect Change/1
  Detect Change/1 -> Chart/1(PulseDetect)
  Chart/1(flag) -> Out1/1
  Constant/1 -> Chart/2(CycleTime)

== system Clutchless_P2_Parallel/Clutchless_HSC/HSC/Camaro Fault Detection/Signal Diagnostic/Transmission Signal Diagnostic/Vehicle Direction Fault Detection ==
  LvrPosTrnsShft : Inport
  Speed : Inport  Port=2
  Compare To Constant : simulink/Logic and Bit Operations/Compare To Constant  relop===  const=4  OutDataTypeStr=boolean
  Compare To Constant1 : simulink/Logic and Bit Operations/Compare To Constant  relop=<  const=0  OutDataTypeStr=boolean
  Compare To Constant2 : simulink/Logic and Bit Operations/Compare To Constant  relop===  const=2  OutDataTypeStr=boolean
  Compare To Constant3 : simulink/Logic and Bit Operations/Compare To Constant  relop=>  const=0  OutDataTypeStr=boolean
  Logical Operator : Logic  AllPortsSameDT=off  OutDataTypeStr=boolean
  Logical Operator1 : Logic  AllPortsSameDT=off  OutDataTypeStr=boolean
  Logical Operator2 : Logic  Operator=OR  AllPortsSameDT=off  OutDataTypeStr=boolean
  Out1 : Outport
  wires:
  LvrPosTrnsShft/1 -> Compare To Constant2/1, Compare To Constant/1
  Speed/1 -> Compare To Constant3/1, Compare To Constant1/1
  Compare To Constant1/1 -> Logical Operator/2
  Compare To Constant/1 -> Logical Operator/1
  Compare To Constant2/1 -> Logical Operator1/1
  Compare To Constant3/1 -> Logical Operator1/2
  Logical Operator1/1 -> Logical Operator2/1
  Logical Operator/1 -> Logical Operator2/2
  Logical Operator2/1 -> Out1/1

== system Clutchless_P2_Parallel/Clutchless_HSC/HSC/Driver_Requests/APP_BPP to DrvIntndAxlTrq2/Post Driver Intnded Axle Torque/Brake Command ==
  APP : Inport
  BPP : Inport  Port=2
  VehicleSpeed : Inport  Port=3
  1-D Lookup Table : Lookup_n-D  NumberOfTableDimensions=1  BreakpointsForDimension1=cal.Regen.BrakeAxleTrq.idx1_BrkPdlPos  Table=cal.Regen.BrakeAxleTrq.map  InternalRulePriority=Speed  RndMeth=Simplest  InputSameDT=on
  Compare To Constant : simulink/Logic and Bit Operations/Compare To Constant  relop=>=  const=cal.Regen.EnableSpeed  OutDataTypeStr=boolean
  Compare To Constant4 : simulink/Logic and Bit Operations/Compare To Constant  relop=<=  const=cal.Regen.EnableAPP  OutDataTypeStr=boolean
  Compare To Constant5 : simulink/Logic and Bit Operations/Compare To Constant  relop=>=  const=cal.Regen.DisableAPP  OutDataTypeStr=boolean
  Constant5 : Constant  Value=0
  Latch : Subsystem
  RegenCal : Gain  Gain=1.3
  Switch : Switch  Criteria=u2 > Threshold  Threshold=1
  Terminator : Terminator
  BrkAxlTrq : Outport
  wires:
  RegenCal/1 -> Switch/1
  Latch/1(Out1) -> Terminator/1
  Compare To Constant4/1 -> Latch/1(Input)
  Compare To Constant5/1 -> Latch/2(Reset)
  Constant5/1 -> Switch/3
  Compare To Constant/1 -> Switch/2
  BPP/1 -> 1-D Lookup Table/1
  APP/1 -> Compare To Constant4/1, Compare To Constant5/1
  Switch/1 -> BrkAxlTrq/1
  1-D Lookup Table/1 -> RegenCal/1
  VehicleSpeed/1 -> Compare To Constant/1

== system Clutchless_P2_Parallel/Clutchless_HSC/HSC/Driver_Requests/APP_BPP to DrvIntndAxlTrq2/Post Driver Intnded Axle Torque/Driver Intended Axle Torque ==
  note: //*mode==1 (CD Mode)
      | mode==2 (CS Mode - Engine Drive)
      | mode==3 (CS Mode-Motor Drive) pass MotTrq
      | mode==4 (Sports Mode) pass Mot Trq+Eng Trq
      | mode==5 (Engine Charging mode)
      | mode==66 (Engine Only mode)*//
  note: In Engine Only mode, ETAS is only as a gateway to broadcast CAN messages
  APP : Inport
  Mode : Inport  Port=2
  TransGearRatio : Inport  Port=3
  Compare To Constant1 : simulink/Logic and Bit Operations/Compare To Constant  relop===  const=2  OutDataTypeStr=boolean
  Compare To Constant2 : simulink/Logic and Bit Operations/Compare To Constant  relop===  const=4  OutDataTypeStr=boolean
  Compare To Constant3 : simulink/Logic and Bit Operations/Compare To Constant  relop===  const=5  OutDataTypeStr=boolean
  Compare To Constant4 : simulink/Logic and Bit Operations/Compare To Constant  relop===  const=1  OutDataTypeStr=boolean
  Compare To Constant5 : simulink/Logic and Bit Operations/Compare To Constant  relop===  const=3  OutDataTypeStr=boolean
  Compare To Constant6 : simulink/Logic and Bit Operations/Compare To Constant  relop===  const=66  OutDataTypeStr=boolean
  Constant : Constant  Value=eng.plant.trq_max_hot_point  VectorParams1D=off
  Constant1 : Constant  Value=fd.plant.init.ratio
  Constant2 : Constant  Value=mot.plant.init.motor.trq_max.points.trq  VectorParams1D=off
  Constant3 : Constant  Value=mot.plant.init.motor.trq_max.points.trq  VectorParams1D=off
  Constant4 : Constant  Value=eng.plant.trq_max_hot_point  VectorParams1D=off
  Gain1 : Gain  Gain=1/100
  Gain2 : Gain  Gain=1/100
  Gain3 : Gain  Gain=1/100
  Logical Operator : Logic  Operator=OR  Inputs=4  AllPortsSameDT=off  OutDataTypeStr=boolean
  Logical Operator1 : Logic  Operator=OR  AllPortsSameDT=off  OutDataTypeStr=boolean
  Memory : Memory
  Product : Product  RndMeth=Zero
  Product1 : Product  RndMeth=Zero
  Product2 : Product  Inputs=3  RndMeth=Zero
  Product3 : Product  RndMeth=Zero
  Ratio Filter : Subsystem
  Sum1 : Sum
  Switch1 : Switch  Threshold=1
  Switch3 : Switch  Threshold=1
  Out1 : Outport
  wires:
  Compare To Constant5/1 -> Logical Operator/4
  Compare To Constant4/1 -> Logical Operator/3
  Compare To Constant6/1 -> Logical Operator1/2
  Logical Operator1/1 -> Switch1/2
  Gain3/1 -> Product3/1
  Constant4/1 -> Product3/2
  APP/1 -> Gain1/1, Gain3/1, Gain2/1
  Memory/1 -> Compare To Constant5/1, Compare To Constant4/1, Compare To Constant1/1, Compare To Constant6/1, Compare To Constant3/1, Compare To Constant2/1
  Compare To Constant3/1 -> Logical Operator1/1
  Switch1/1 -> Product2/1
  Product3/1 -> Switch1/1, [IntdAxleTrq_eng]
  Logical Operator/1 -> Switch3/2
  Switch3/1 -> Switch1/3  "DrvIntndAxlTrq"
  Constant/1 -> Sum1/2
  Compare To Constant2/1 -> Logical Operator/2
  Sum1/1 -> Product/1
  Compare To Constant1/1 -> Logical Operator/1
  Constant3/1 -> Sum1/1
  Gain1/1 -> Product/2
  Product2/1 -> Out1/1  "DrvIntndAxlTrq"
  TransGearRatio/1 -> Ratio Filter/1(Ratio)
  Product1/1 -> Switch3/3
  Constant1/1 -> Product2/3  "ratio"
  Mode/1 -> Memory/1
  Product/1 -> Switch3/1
  Gain2/1 -> Product1/2
  Ratio Filter/1(Filtered_Ratio) -> Product2/2
  Constant2/1 -> Product1/1

== system Clutchless_P2_Parallel/Clutchless_HSC/HSC/Powertrain Manager/HV Manager/BMS_Manager/Fault Latch ==
  IsoFault : Inport
  Off Delay : powerlib_meascontrol/Logic/On Delay  DelayType=Off delay  delay=3  ic=0  Ts=0
      settings: SourceProductName=Simscape Power Systems
  IsoFaultLatched : Outport
  wires:
  Off Delay/1 -> IsoFaultLatched/1
  IsoFault/1 -> Off Delay/1

== system Clutchless_P2_Parallel/Clutchless_HSC/HSC/Powertrain Manager/HV Manager/BMS_Manager/ISO_Hybrid_01_Req ==
  In1 : Inport
  Bus Creator : BusCreator  Inputs=9
  ISO_Hybrid_01_Req_Data_byte_0 : Constant  Value=3
  ISO_Hybrid_01_Req_Data_byte_1 : Constant  Value=34
  ISO_Hybrid_01_Req_Data_byte_2 : Constant  Value=30
  ISO_Hybrid_01_Req_Data_byte_3 : Constant  Value=25
  ISO_Hybrid_01_Req_Data_byte_{4..7} (4 alike) : Constant  Value=0
  ISO_Hybrid_01_Req_Data_byte_8 : Constant  Value=23
  ISO_Request : DiscretePulseGenerator  PulseType=Time based  Period=0.5  PulseWidth=50  SampleTime=-1
  Switch{,1..8} (9 alike) : Switch  Criteria=u2 > Threshold
  Out1 : Outport
  wires:
  ISO_Request/1 -> Switch/2  "<ISO_Hybrid_01_Req_Data_byte_3>"
  ISO_Hybrid_01_Req_Data_byte_7/1 -> Switch8/1
  ISO_Hybrid_01_Req_Data_byte_6/1 -> Switch7/1
  ISO_Hybrid_01_Req_Data_byte_5/1 -> Switch6/1
  ISO_Hybrid_01_Req_Data_byte_4/1 -> Switch5/1
  Switch/1 -> Switch4/1  "ISO_Hybrid_01_Req_Data_byte_3"
  ISO_Hybrid_01_Req_Data_byte_2/1 -> Switch3/1
  ISO_Hybrid_01_Req_Data_byte_1/1 -> Switch2/1
  In1/1 -> Switch1/2, Switch1/3, Switch2/3, Switch3/2, Switch4/2, Switch5/2, Switch6/2, Switch8/3, Bus Creator/9, Switch8/2, Switch7/3, Switch7/2, Switch6/3, Switch5/3, Switch4/3, Switch3/3, Switch2/2
  ISO_Hybrid_01_Req_Data_byte_0/1 -> Switch1/1
  Switch4/1 -> Bus Creator/4  "ISO_Hybrid_01_Req_Data_byte_3"
  Switch8/1 -> Bus Creator/8  "ISO_Hybrid_01_Req_Data_byte_7"
  Switch2/1 -> Bus Creator/2  "ISO_Hybrid_01_Req_Data_byte_1"
  Switch7/1 -> Bus Creator/7  "ISO_Hybrid_01_Req_Data_byte_6"
  Switch1/1 -> Bus Creator/1  "ISO_Hybrid_01_Req_Data_byte_0"
  ISO_Hybrid_01_Req_Data_byte_3/1 -> Switch/1
  Switch3/1 -> Bus Creator/3  "ISO_Hybrid_01_Req_Data_byte_2"
  Switch5/1 -> Bus Creator/5  "ISO_Hybrid_01_Req_Data_byte_4"
  ISO_Hybrid_01_Req_Data_byte_8/1 -> Switch/3
  Switch6/1 -> Bus Creator/6  "ISO_Hybrid_01_Req_Data_byte_5"
  Bus Creator/1 -> Out1/1  "ISO_Hybrid_01_Req"
